simulink model "lab3csim"  (R2023a)
settings: Solver=FixedStepAuto  StartTime=0.0  StopTime=1  FixedStep=1/1024  RelTol=1e-3
values from neighbouring files (symbols this model uses):
  N = 10    [lab3a_script.m]
undefined symbols (not defined in the file or in its folder): r2r
settings Model: Creator=a96an  LastModifiedBy=a96an
settings DataIOCC: ReturnWorkspaceOutputs=off

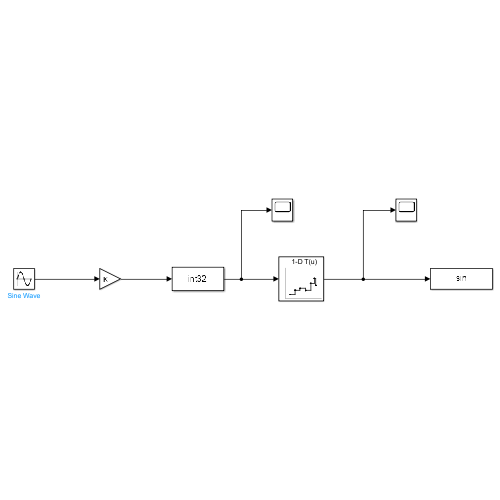
[thumbnail: Simulink's stored preview of the top-level diagram]
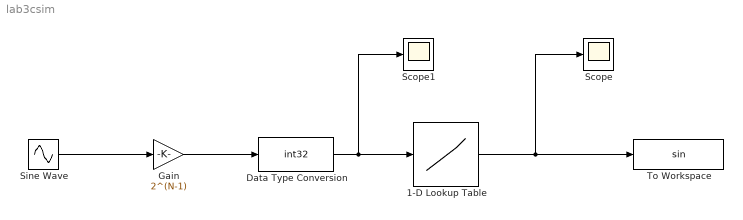
== system lab3csim ==
  1-D Lookup Table : Lookup_n-D  NumberOfTableDimensions=1  BreakpointsForDimension1=-2^(N-1):(2^(N-1))-1  Table=r2r(N)  InterpMethod=Flat  InternalRulePriority=Speed  OutDataTypeStr=double  RndMeth=Simplest
  Data Type Conversion : DataTypeConversion  OutDataTypeStr=int32  RndMeth=Nearest  SaturateOnIntegerOverflow=off
  Gain : Gain  Gain=2^(N-1)
  Scope : Scope
  Scope1 : Scope
  Sine Wave : Sin  Frequency=2*pi*5  SampleTime=0
  To Workspace : ToWorkspace  VariableName=sin  SaveFormat=Timeseries  SampleTime=-1
  wires:
  1-D Lookup Table/1 -> Scope/1, To Workspace/1
  Data Type Conversion/1 -> Scope1/1, 1-D Lookup Table/1
  Gain/1 -> Data Type Conversion/1
  Sine Wave/1 -> Gain/1
